simulink subsystem "Controlador"  (R2023b)
settings: Solver=VariableStepAuto  StartTime=0.0  StopTime=10.0  RelTol=1e-3
settings Model: Creator=chaya  LastModifiedBy=chaya

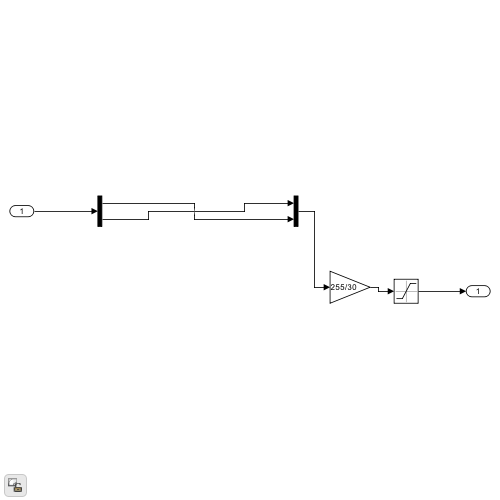
[thumbnail: Simulink's stored preview of the top-level diagram]
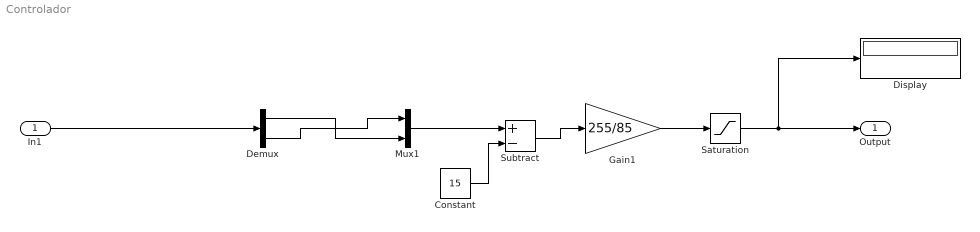
== system Controlador ==
  In1 : Inport
  Constant : Constant  Value=15
  Demux : Demux  Outputs=2
  Display : Display
  Gain1 : Gain  Gain=255/85
  Mux1 : Mux  Inputs=2
  Saturation : Saturate  UpperLimit=100  LowerLimit=-100
  Subtract : Sum  Inputs=+-
  Output : Outport
  wires:
  Demux/2 -> Mux1/1
  Demux/1 -> Mux1/2
  Gain1/1 -> Saturation/1
  Mux1/1 -> Subtract/1
  Subtract/1 -> Gain1/1
  Constant/1 -> Subtract/2
  In1/1 -> Demux/1
  Saturation/1 -> Output/1, Display/1
